simulink model "TestWalsh03Class_home"  (R2021a)
settings: Solver=VariableStepAuto  StartTime=0.0  StopTime=96  RelTol=1e-3
settings Model: Creator=alexandr.lanin  LastModifiedBy=Alex
settings SolverCC: AlgebraicLoopSolver=TrustRegion
settings DataIOCC: ReturnWorkspaceOutputs=off
settings DebuggingCC: SFMachineParentedDataDiag=warning  ArithmeticOperatorsInVariantConditions=warning
settings SFSimCC: SimUseLocalCustomCode=off  CustomCodeUndefinedFunction=UseInterfaceOnly
settings RTWCC: RTWUseLocalCustomCode=off
settings CodeAppCC: StateflowObjectComments=on

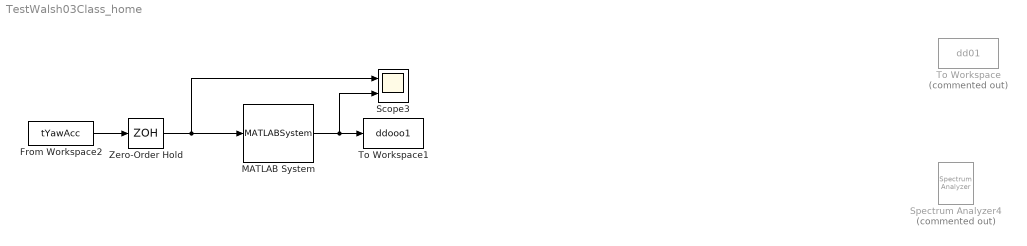
== system TestWalsh03Class_home ==
  From Workspace2 : FromWorkspace  VariableName=tYawAcc
  MATLAB System : MATLABSystem  System=WolchSim  SimulateUsing=Code generation
      mask Type: WolchSim
      mask Display:
      | disp('WolchSim');
      | port_label('input',1,'u');
      | port_label('output',1,'y');
  Scope3 : Scope  NumInputPorts=2
  Spectrum Analyzer4 : SpectrumAnalyzer  Commented=on
  To Workspace : ToWorkspace  Commented=on  VariableName=dd01  SaveFormat=Timeseries  SampleTime=-1
  To Workspace1 : ToWorkspace  VariableName=ddooo1  SaveFormat=Timeseries  SampleTime=-1
  Zero-Order Hold : ZeroOrderHold  SampleTime=0.01
  wires:
  From Workspace2/1 -> Zero-Order Hold/1
  MATLAB System/1 -> Scope3/2, To Workspace1/1
  Zero-Order Hold/1 -> Scope3/1, MATLAB System/1
